simulink model "simulink2"  (R2018a)
settings: Solver=VariableStepAuto  StartTime=0.0  StopTime=10.0  RelTol=1e-3
settings Model: Creator=Surja Kamal Ghosh  LastModifiedBy=Surja Kamal Ghosh

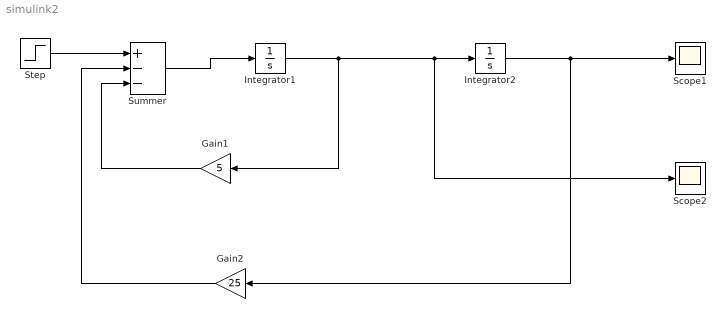
== system simulink2 ==
  Gain1 : Gain  Gain=5
  Gain2 : Gain  Gain=25
  Integrator1 : Integrator
  Integrator2 : Integrator  ContinuousStateAttributes=Scope1
  Scope1 : Scope
  Scope2 : Scope
  Step : Step  After=25  SampleTime=0
  Summer : Sum  Inputs=+--
  wires:
  Gain1/1 -> Summer/3
  Step/1 -> Summer/1
  Summer/1 -> Integrator1/1
  Integrator1/1 -> Gain1/1, Scope2/1, Integrator2/1
  Integrator2/1 -> Gain2/1, Scope1/1
  Gain2/1 -> Summer/2
